simulink model "computeG"  (Simulink 7.9)
settings: Solver=FixedStepDiscrete  StartTime=0.0  StopTime=960  FixedStep=Ts  RelTol=1e-3
InitFcn:
  | robotName = 'icubGazeboSim';
  | localName = 'SimulinkiCubGazeboSim';
  | Ts = 0.1;
libraries: WBCLibrary x8, simulink x1
settings Model: Creator=iron  LastModifiedBy=jorhabib
settings DebuggingCC: FcnCallInpInsideContextMsg=Use local settings
settings CodeAppCC: CustomSymbolStrType=$N$R$M_T
settings GRTTargetCC: CodeReplacementLibrary=C89/C90 (ANSI)  CombineOutputUpdateFcns=off  GRTInterface=on

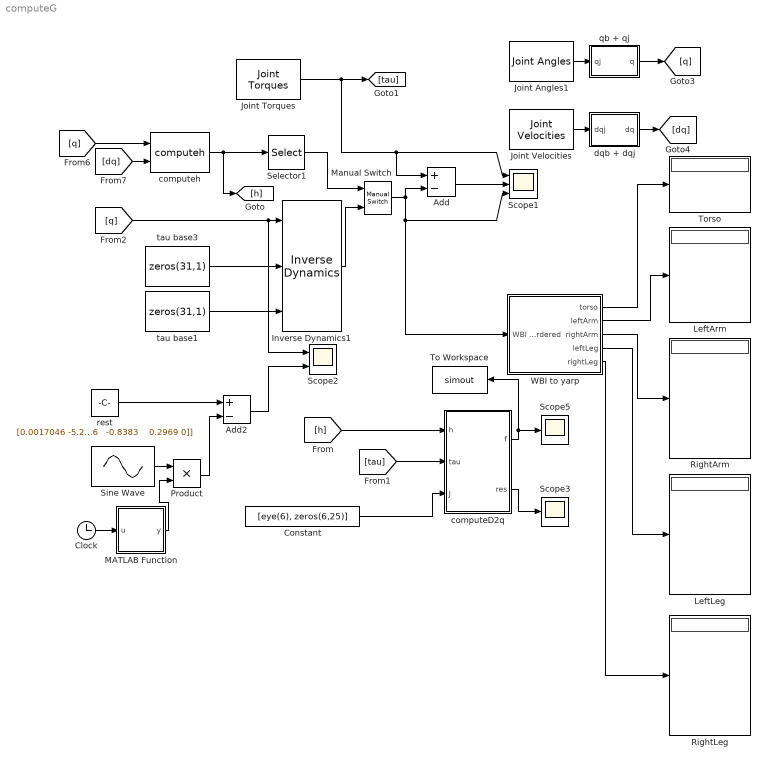
== system computeG ==
  Add : Sum  Inputs=+-
  Add2 : Sum  Inputs=+-
  Clock : Clock
  Constant : Constant  Value=[eye(6), zeros(6,25)]  VectorParams1D=off
  Inverse Dynamics1 : WBCLibrary/wholeBodyModel/Dynamics/Inverse Dynamics  robotName=robotName  localName=localName
  Joint Angles1 : WBCLibrary/wholeBodyStates/Joint Angles  robotName=robotName  localName=localName
  Joint Torques : WBCLibrary/wholeBodyStates/Joint Torques  robotName=robotName  localName=localName
  Joint Velocities : WBCLibrary/wholeBodyStates/Joint Velocities  robotName=robotName  localName=localName
  LeftArm : Display
  LeftLeg : Display
  MATLAB Function : MATLAB Function  TreatAsAtomicUnit=on
      settings: PermitHierarchicalResolution=ParametersOnly
  Manual Switch : simulink/Signal Routing/Manual Switch  sw=0  action=0  varsize=off
  Product : Product  RndMeth=Zero
  RightArm : Display
  RightLeg : Display
  Scope1 : Scope  NumInputPorts=3
      settings: TimeRange=600  YMin=-15~-5~-15  YMax=5~10~5
  Scope2 : Scope  NumInputPorts=2
      settings: TimeRange=10  YMin=-0.6~-0.9  YMax=0.8~1
  Scope3 : Scope
      settings: YMin=-0.025  YMax=0.05  SaveName=ScopeData3
  Scope5 : Scope
      settings: YMax=10  SaveName=ScopeData2
  Selector1 : Selector  InputPortWidth=31  Indices=[7:31]
  Sine Wave : Sin  Amplitude=0.2  Bias=-0.2  Frequency=.05/2*pi  Phase=pi/2  Samples=100  SampleTime=Ts
  To Workspace : ToWorkspace  VariableName=simout  SaveFormat=Structure  SampleTime=-1
  Torso : Display
  WBI to yarp : Subsystem
  computeD2q : MATLAB Function  TreatAsAtomicUnit=on
      settings: PermitHierarchicalResolution=ParametersOnly
  computeh : WBCLibrary/wholeBodyModel/Dynamics/computeh  val=7  robotname=robotName  localname=localName
  dqb + dqj : Subsystem
  qb + qj : Subsystem
  rest : Constant  Value="[0.0017046 -5.2083e-07  1.5067e-06    -0.51794     0.51843  0.00024936     0.78334 -8.2867e-05    -0.51794     0.51843   0.0002485     0.78334  -8.263e-05 [0.6854    0.8055    0.0026   -0.8383    0.2969 0]  [0.6854    0.8055    0.0026   -0.8383    0.2969 0]]"
  tau base1 : Constant  Value=zeros(31,1)
  tau base3 : Constant  Value=zeros(31,1)
  wires:
  [q] -> Inverse Dynamics1/1, Scope2/1
  tau base3/1 -> Inverse Dynamics1/2
  tau base1/1 -> Inverse Dynamics1/3
  computeh/1 -> Selector1/1, [h]
  Add2/1 -> Scope2/2
  Add/1 -> Scope1/2
  rest/1 -> Add2/1
  Sine Wave/1 -> Product/1
  Joint Torques/1 -> [tau], Scope1/1, Add/1
  WBI to yarp/1(torso) -> Torso/1
  WBI to yarp/2(leftArm) -> LeftArm/1
  WBI to yarp/3(rightArm) -> RightArm/1
  WBI to yarp/4(leftLeg) -> LeftLeg/1
  WBI to yarp/5(rightLeg) -> RightLeg/1
  Product/1 -> Add2/2
  Clock/1 -> MATLAB Function/1(u)
  MATLAB Function/1(y) -> Product/2
  [tau] -> computeD2q/2(tau)
  Constant/1 -> computeD2q/3(J)
  computeD2q/2(res) -> Scope3/1
  computeD2q/1(f) -> Scope5/1, To Workspace/1
  [h] -> computeD2q/1(h)
  Joint Angles1/1 -> qb + qj/1(qj)
  qb + qj/1(q) -> [q]
  [q] -> computeh/1
  [dq] -> computeh/2
  Joint Velocities/1 -> dqb + dqj/1(dqj)
  dqb + dqj/1(dq) -> [dq]
  Manual Switch/1 -> Add/2, WBI to yarp/1(WBI ordered), Scope1/3
  Selector1/1 -> Manual Switch/1
  Inverse Dynamics1/1 -> Manual Switch/2

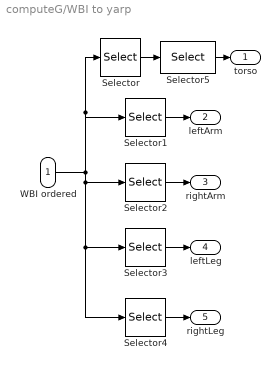
== system computeG/WBI to yarp ==
  WBI ordered : Inport
  Selector : Selector  InputPortWidth=25  Indices=[1 2 3]
  Selector1 : Selector  InputPortWidth=25  Indices=[4 5 6 7 8]
  Selector2 : Selector  InputPortWidth=25  Indices=[9 10 11 12 13]
  Selector3 : Selector  InputPortWidth=25  Indices=[14 15 16 17 18 19]
  Selector4 : Selector  InputPortWidth=25  Indices=[20 21 22 23 24 25]
  Selector5 : Selector  InputPortWidth=3  Indices=[3 2 1]
  torso : Outport
  leftArm : Outport  Port=2
  rightArm : Outport  Port=3
  leftLeg : Outport  Port=4
  rightLeg : Outport  Port=5
  wires:
  Selector1/1 -> leftArm/1
  Selector2/1 -> rightArm/1
  Selector3/1 -> leftLeg/1
  Selector4/1 -> rightLeg/1
  WBI ordered/1 -> Selector/1, Selector1/1, Selector2/1, Selector4/1, Selector3/1
  Selector/1 -> Selector5/1
  Selector5/1 -> torso/1

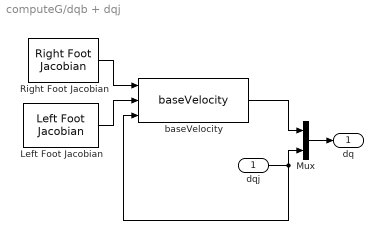
== system computeG/dqb + dqj ==
  dqj : Inport
  Left Foot Jacobian : WBCLibrary/wholeBodyModel/Jacobians/Left Foot Jacobian  robotName=robotName  localName=localName
  Mux : Mux  Inputs=2
  Right Foot Jacobian : WBCLibrary/wholeBodyModel/Jacobians/Right Foot Jacobian  robotName=robotName  localName=localName
  baseVelocity : WBCLibrary/Utilities/baseVelocity
  dq : Outport
  wires:
  Left Foot Jacobian/1 -> baseVelocity/2
  Right Foot Jacobian/1 -> baseVelocity/1
  baseVelocity/1 -> Mux/1
  dqj/1 -> baseVelocity/3, Mux/2
  Mux/1 -> dq/1

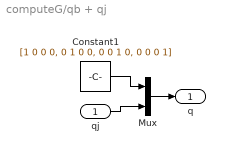
== system computeG/qb + qj ==
  qj : Inport
  Constant1 : Constant  Value=[1 0 0 0, 0 1 0 0, 0 0 1 0, 0 0 0 1]
  Mux : Mux  Inputs=2
  q : Outport
  wires:
  Mux/1 -> q/1
  Constant1/1 -> Mux/1
  qj/1 -> Mux/2

== matlab function computeD2q ==
  data: h input double; tau input double; J input double; f output double; res output double
function [f, res] = fcn(h, tau, J)

% Francesco Nori
% Genova 10 Marzo 2014
% CODYCO project
%
% This code computes the d2q given the currently applied torques,
% assuming contacts at both feet.
%
% M d2q + h - J' f = S' tau  
%
% with the constraints being described as:
%
% J dq = 0
%
% J d2q + dJdq= 0

[~, n] = size(J);
S = [zeros(n-6, 6), eye(n-6)];
f = -pinv(J')*(S'*tau - h);
res = J'*f + S'*tau - h;

% res = h(7:31) - tau;
% f = 0;

== matlab function MATLAB Function ==
  data: u input double; y output double
function y = fcn(u)
%#codegen

y = zeros(25,1);
index = floor(u/80) + 14;
if index > 0 && index < 26
    y(index) = 1;
end
